simulink model "Motor_pos"  (R2020b)
settings: Solver=VariableStepAuto  StartTime=0.0  StopTime=10.0  RelTol=1e-3
settings Model: Creator=MY lenovo  LastModifiedBy=MY lenovo
settings DataIOCC: SaveOutput=off  SaveTime=off

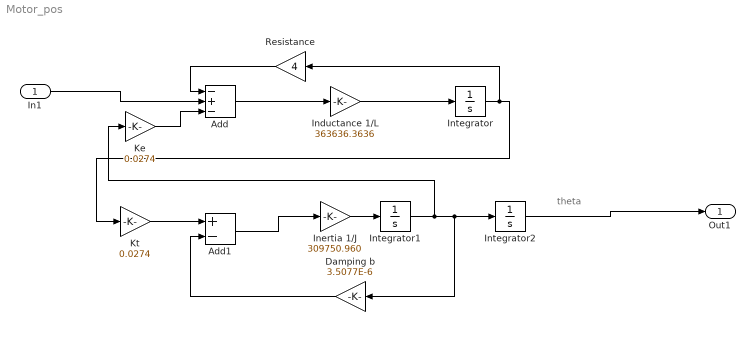
== system Motor_pos ==
  note: theta
  In1 : Inport  OutDataTypeStr=double  PortDimensions=1  SampleTime=0
  Add : Sum  Inputs=-+-
  Add1 : Sum  Inputs=+-
  Damping b : Gain  Gain=3.5077E-6
  Inductance 1/L : Gain  Gain=363636.3636
  Inertia 1/J : Gain  Gain=309750.960
  Integrator : Integrator
  Integrator1 : Integrator
  Integrator2 : Integrator
  Ke : Gain  Gain=0.0274
  Kt : Gain  Gain=0.0274
  Resistance : Gain  Gain=4
  Out1 : Outport  OutDataTypeStr=double  PortDimensions=1  SampleTime=0
  wires:
  Add/1 -> Inductance 1/L/1
  Resistance/1 -> Add/1
  Kt/1 -> Add1/1
  Inductance 1/L/1 -> Integrator/1
  Ke/1 -> Add/3
  Inertia 1/J/1 -> Integrator1/1
  Integrator/1 -> Kt/1, Resistance/1
  Damping b/1 -> Add1/2
  Integrator1/1 -> Integrator2/1, Damping b/1, Ke/1
  Add1/1 -> Inertia 1/J/1
  Integrator2/1 -> Out1/1
  In1/1 -> Add/2
